simulink model "E33_VCU_simulink"  (R2014a)
settings: Solver=FixedStepDiscrete  StartTime=0.0  StopTime=10.0  FixedStep=0.0005  RelTol=1e-3
values from neighbouring files (symbols this model uses):
  Accu_FAN_Test = ecucoder_cal(Accu_FAN_Test)    [E33_VCU.m]
  Accu_FAN_threshold = ecucoder_cal(Accu_FAN_threshold)    [E33_VCU.m]
  APPS1_Voltage = ecucoder_cal(APPS1_Voltage)    [E33_VCU.m]
  APPS2_Voltage = ecucoder_cal(APPS2_Voltage)    [E33_VCU.m]
  APPS_Map = [0,1000]    [E33_VCU.m]
  APPS_threshold = ecucoder_cal(APPS_threshold)    [E33_VCU.m]
  Beep_Time = ecucoder_cal(Beep_Time)    [E33_VCU.m]
  BeeperTest = ecucoder_cal(BeeperTest)    [E33_VCU.m]
  BMSLedTest = ecucoder_cal(BMSLedTest)    [E33_VCU.m]
  BP_F_threshold = ecucoder_cal(BP_F_threshold)    [E33_VCU.m]
  BP_F_Voltage = ecucoder_cal(BP_F_Voltage)    [E33_VCU.m]
  BP_Map = [0,1000]    [E33_VCU.m]
  BP_R_Voltage = ecucoder_cal(BP_R_Voltage)    [E33_VCU.m]
  Brk_luminance = ecucoder_cal(Brk_luminance)    [E33_VCU.m]
  DCDC_Relay_Test = ecucoder_cal(DCDC_Relay_Test)    [E33_VCU.m]
  FactoryTestEnable = ecucoder_cal(FactoryTestEnable)    [E33_VCU.m]
  HardBrk_luminance = ecucoder_cal(HardBrk_luminance)    [E33_VCU.m]
  IMDLedTest = ecucoder_cal(IMDLedTest)    [E33_VCU.m]
  linear_FL_Map = ecucoder_cal(linear_FL_Map)    [E33_VCU.m]
  linear_FR_Map = ecucoder_cal(linear_FR_Map)    [E33_VCU.m]
  linear_Map = ecucoder_cal(linear_Map)    [E33_VCU.m]
  linear_RL_Map = ecucoder_cal(linear_RL_Map)    [E33_VCU.m]
  linear_RR_Map = ecucoder_cal(linear_RR_Map)    [E33_VCU.m]
  MaxPow = 40    [E33_VCU.m]
  MaxRPM = 5400    [E33_VCU.m]
  MaxRPMchangePerSec = ecucoder_cal(MaxRPMchangePerSec)    [E33_VCU.m]
  MaxTorqChangePerSec = ecucoder_cal(MaxTorqChangePerSec)    [E33_VCU.m]
  Motor_RPM_Map = (0:ceil(MaxRPM/100))*100    [E33_VCU.m]
  Pump_Test = ecucoder_cal(Pump_Test)    [E33_VCU.m]
  Pump_threshold = ecucoder_cal(Pump_threshold)    [E33_VCU.m]
  R2D_Light_Test = ecucoder_cal(R2D_Light_Test)    [E33_VCU.m]
  Radiator_FAN_Test = ecucoder_cal(Radiator_FAN_Test)    [E33_VCU.m]
  SCS_Error_5V = ecucoder_cal(SCS_Error_5V)    [E33_VCU.m]
  SCS_Error_GND = ecucoder_cal(SCS_Error_GND)    [E33_VCU.m]
  SPD_Coef = 1884/40    (= 47.1)    [E33_VCU.m]
  Tail_Light_Test = ecucoder_cal(Tail_Light_Test)    [E33_VCU.m]
  Tmanage_Map = [0,100]    [E33_VCU.m]
  Torq_percentage_Map = Motor_Torq_MAP/MaxTorq*1000    [E33_VCU.m]
libraries: simulink x164, ec55xxlib x44, dspswit3 x6
(part 2 of 5)

== system E33_VCU_simulink/Input/Input/Sensor ==
  function : TriggerPort  TriggerType=function-call
  1-D Lookup Table1 : Lookup_n-D  NumberOfTableDimensions=1  BreakpointsForDimension1=linear_RR_Map  Table=linear_Map  ExtrapMethod=Clip  InternalRulePriority=Speed  OutDataTypeStr=uint16  RndMeth=Simplest  InputSameDT=on
  1-D Lookup Table2 : Lookup_n-D  NumberOfTableDimensions=1  BreakpointsForDimension1=linear_FR_Map  Table=linear_Map  ExtrapMethod=Clip  InternalRulePriority=Speed  OutDataTypeStr=uint16  RndMeth=Simplest  InputSameDT=on
  1-D Lookup Table3 : Lookup_n-D  NumberOfTableDimensions=1  BreakpointsForDimension1=linear_RL_Map  Table=linear_Map  ExtrapMethod=Clip  InternalRulePriority=Speed  OutDataTypeStr=uint16  RndMeth=Simplest  InputSameDT=on
  1-D Lookup Table4 : Lookup_n-D  NumberOfTableDimensions=1  BreakpointsForDimension1=linear_FL_Map  Table=linear_Map  ExtrapMethod=Clip  InternalRulePriority=Speed  OutDataTypeStr=uint16  RndMeth=Simplest  InputSameDT=on
  1-D Lookup Table5 : Lookup_n-D  NumberOfTableDimensions=1  BreakpointsForDimension1=[500,900,2007,2205,3405,3705,4490]  BreakpointsForDimension1DataTypeStr=int32  Table=[-364,0,1000,1000,-1000,-1000,-365]  TableDataTypeStr=int32  IntermediateResultsDataTypeStr=int32  ExtrapMethod=Clip  InternalRulePriority=Speed  OutDataTypeStr=int32  RndMeth=Simplest  InputSameDT=on
  AnalogInput : ec55xxlib/RapidECU_U2/02AnalogInput/AnalogInput  channel=56: I_AN17_5V  sampletime=-1
  AnalogInput1 : ec55xxlib/RapidECU_U2/02AnalogInput/AnalogInput  channel=71: I_AN18_5V  sampletime=-1
  AnalogInput2 : ec55xxlib/RapidECU_U2/02AnalogInput/AnalogInput  channel=73: I_AN19_5V  sampletime=-1
  AnalogInput3 : ec55xxlib/RapidECU_U2/02AnalogInput/AnalogInput  channel=74: I_AN20_5V  sampletime=-1
  AnalogInput4 : ec55xxlib/RapidECU_U2/02AnalogInput/AnalogInput  channel=14: I_AN04_2K55  sampletime=-1
  Constant : Constant  Commented=on  Value=SPD_Coef
  Data Type Conversion{,1..3} (4 alike) : DataTypeConversion  Commented=on  OutDataTypeStr=double
  Demux : Demux  Commented=on
  Filter1 : Subsystem
  Filter2 : Subsystem
  Filter3 : Subsystem
  Filter4 : Subsystem
  For Each Subsystem : Subsystem  Commented=on  TreatAsAtomicUnit=on
  FrequencyRead : ec55xxlib/RapidECU_U2/03FrequencyInput/FrequencyRead  Commented=on  channel=41: I_HALL5  sampletime=-1
  FrequencyRead1 : ec55xxlib/RapidECU_U2/03FrequencyInput/FrequencyRead  Commented=on  channel=38: I_HALL2  sampletime=-1
  FrequencyRead2 : ec55xxlib/RapidECU_U2/03FrequencyInput/FrequencyRead  Commented=on  channel=39: I_HALL3  sampletime=-1
  FrequencyRead3 : ec55xxlib/RapidECU_U2/03FrequencyInput/FrequencyRead  Commented=on  channel=40: I_HALL4  sampletime=-1
  Mux : Mux  Commented=on
  Linear_RR : Outport
  Linear_FR : Outport  Port=2
  Linear_RL : Outport  Port=3
  Linear_FL : Outport  Port=4
  Wheel_Angle : Outport  Port=5
  wires:
  AnalogInput3/1 -> Filter4/1(In)
  AnalogInput2/1 -> Filter2/1(In)
  AnalogInput1/1 -> Filter1/1(In)
  AnalogInput/1 -> Filter3/1(In)
  AnalogInput4/1 -> 1-D Lookup Table5/1  "Angle_Vol"
  Filter3/1(Out) -> 1-D Lookup Table1/1
  1-D Lookup Table1/1 -> Linear_RR/1
  Filter1/1(Out) -> 1-D Lookup Table2/1
  1-D Lookup Table2/1 -> Linear_FR/1
  Filter2/1(Out) -> 1-D Lookup Table3/1
  1-D Lookup Table3/1 -> Linear_RL/1
  Filter4/1(Out) -> 1-D Lookup Table4/1
  1-D Lookup Table4/1 -> Linear_FL/1
  1-D Lookup Table5/1 -> Wheel_Angle/1
  FrequencyRead1/1 -> Mux/1  "SPD_RR_Vol"
  FrequencyRead2/1 -> Mux/2  "SPD_FR_Voll"
  FrequencyRead3/1 -> Mux/3
  FrequencyRead/1 -> Mux/4
  Mux/1 -> For Each Subsystem/1(In1)
  Constant/1 -> For Each Subsystem/2(In2)
  For Each Subsystem/1(Out1) -> Demux/1
  Demux/1 -> Data Type Conversion/1  "SPD_RR"
  Demux/2 -> Data Type Conversion1/1  "SPD_FR"
  Demux/3 -> Data Type Conversion2/1  "SPD_RL"
  Demux/4 -> Data Type Conversion3/1  "SPD_FL"
  Data Type Conversion/1 -> ?
  Data Type Conversion1/1 -> ?
  Data Type Conversion2/1 -> ?
  Data Type Conversion3/1 -> ?

== system E33_VCU_simulink/Subsystem1/MCUctrl/MCU_CMD_CAN_Tx ==
  Msg : Inport
  Enable : EnablePort
  CANTransmit : ec55xxlib/RapidECU_U2/07CANCommucation/CANTransmit  canmodule=A  canbuffer=8  canmessageid=hex2dec('08C1EF21')  canmessagetype=Extended(29-bit ID)  datalength=8  sampletime=-1
  CAN_OK : Outport
  wires:
  Msg/1 -> CANTransmit/1
  CANTransmit/1 -> CAN_OK/1  "VCUMCUCANOKK"

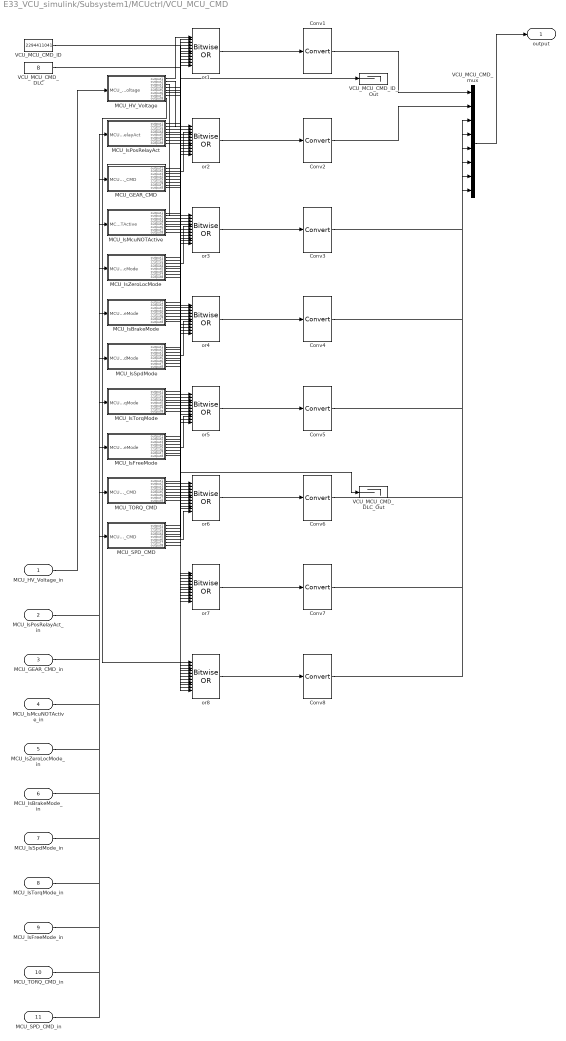
== system E33_VCU_simulink/Subsystem1/MCUctrl/VCU_MCU_CMD ==
  MCU_HV_Voltage_in : Inport
  MCU_IsPosRelayAct_in : Inport  Port=2
  MCU_GEAR_CMD_in : Inport  Port=3
  MCU_IsMcuNOTActive_in : Inport  Port=4
  MCU_IsZeroLocMode_in : Inport  Port=5
  MCU_IsBrakeMode_in : Inport  Port=6
  MCU_IsSpdMode_in : Inport  Port=7
  MCU_IsTorqMode_in : Inport  Port=8
  MCU_IsFreeMode_in : Inport  Port=9
  MCU_TORQ_CMD_in : Inport  Port=10
  MCU_SPD_CMD_in : Inport  Port=11
  Conv{1..8} (8 alike) : DataTypeConversion
  MCU_GEAR_CMD : Subsystem
  MCU_HV_Voltage : Subsystem
  MCU_IsBrakeMode : Subsystem
  MCU_IsFreeMode : Subsystem
  MCU_IsMcuNOTActive : Subsystem
  MCU_IsPosRelayAct : Subsystem
  MCU_IsSpdMode : Subsystem
  MCU_IsTorqMode : Subsystem
  MCU_IsZeroLocMode : Subsystem
  MCU_SPD_CMD : Subsystem
  MCU_TORQ_CMD : Subsystem
  VCU_MCU_CMD_DLC : Constant  Value=8  OutDataTypeStr=uint8
  VCU_MCU_CMD_DLC_Out : Terminator
  VCU_MCU_CMD_ID : Constant  Value=2294411041  OutDataTypeStr=single
  VCU_MCU_CMD_ID_Out : Terminator
  VCU_MCU_CMD_mux : Mux  Inputs=8
  or{1..8} (8 alike) : simulink/Logic and Bit Operations/Bitwise Operator  logicop=OR  UseBitMask=off  NumInputPorts=11  BitMask=bin2dec('11011001')  BitMaskRealWorld=Stored Integer
  output : Outport
  wires:
  VCU_MCU_CMD_mux/1 -> output/1
  MCU_HV_Voltage/1(output1) -> or1/1
  MCU_HV_Voltage/2(output2) -> or2/1
  MCU_HV_Voltage/3(output3) -> or3/1
  MCU_HV_Voltage/4(output4) -> or4/1
  MCU_HV_Voltage/5(output5) -> or5/1
  MCU_HV_Voltage/6(output6) -> or6/1
  MCU_HV_Voltage/7(output7) -> or7/1
  MCU_HV_Voltage/8(output8) -> or8/1
  MCU_IsPosRelayAct/1(output1) -> or1/2
  MCU_IsPosRelayAct/2(output2) -> or2/2
  MCU_IsPosRelayAct/3(output3) -> or3/2
  MCU_IsPosRelayAct/4(output4) -> or4/2
  MCU_IsPosRelayAct/5(output5) -> or5/2
  MCU_IsPosRelayAct/6(output6) -> or6/2
  MCU_IsPosRelayAct/7(output7) -> or7/2
  MCU_IsPosRelayAct/8(output8) -> or8/2
  MCU_GEAR_CMD/1(output1) -> or1/3
  MCU_GEAR_CMD/2(output2) -> or2/3
  MCU_GEAR_CMD/3(output3) -> or3/3
  MCU_GEAR_CMD/4(output4) -> or4/3
  MCU_GEAR_CMD/5(output5) -> or5/3
  MCU_GEAR_CMD/6(output6) -> or6/3
  MCU_GEAR_CMD/7(output7) -> or7/3
  MCU_GEAR_CMD/8(output8) -> or8/3
  MCU_IsMcuNOTActive/1(output1) -> or1/4
  MCU_IsMcuNOTActive/2(output2) -> or2/4
  MCU_IsMcuNOTActive/3(output3) -> or3/4
  MCU_IsMcuNOTActive/4(output4) -> or4/4
  MCU_IsMcuNOTActive/5(output5) -> or5/4
  MCU_IsMcuNOTActive/6(output6) -> or6/4
  MCU_IsMcuNOTActive/7(output7) -> or7/4
  MCU_IsMcuNOTActive/8(output8) -> or8/4
  MCU_IsZeroLocMode/1(output1) -> or1/5
  MCU_IsZeroLocMode/2(output2) -> or2/5
  MCU_IsZeroLocMode/3(output3) -> or3/5
  MCU_IsZeroLocMode/4(output4) -> or4/5
  MCU_IsZeroLocMode/5(output5) -> or5/5
  MCU_IsZeroLocMode/6(output6) -> or6/5
  MCU_IsZeroLocMode/7(output7) -> or7/5
  MCU_IsZeroLocMode/8(output8) -> or8/5
  MCU_IsBrakeMode/1(output1) -> or1/6
  MCU_IsBrakeMode/2(output2) -> or2/6
  MCU_IsBrakeMode/3(output3) -> or3/6
  MCU_IsBrakeMode/4(output4) -> or4/6
  MCU_IsBrakeMode/5(output5) -> or5/6
  MCU_IsBrakeMode/6(output6) -> or6/6
  MCU_IsBrakeMode/7(output7) -> or7/6
  MCU_IsBrakeMode/8(output8) -> or8/6
  MCU_IsSpdMode/1(output1) -> or1/7
  MCU_IsSpdMode/2(output2) -> or2/7
  MCU_IsSpdMode/3(output3) -> or3/7
  MCU_IsSpdMode/4(output4) -> or4/7
  MCU_IsSpdMode/5(output5) -> or5/7
  MCU_IsSpdMode/6(output6) -> or6/7
  MCU_IsSpdMode/7(output7) -> or7/7
  MCU_IsSpdMode/8(output8) -> or8/7
  MCU_IsTorqMode/1(output1) -> or1/8
  MCU_IsTorqMode/2(output2) -> or2/8
  MCU_IsTorqMode/3(output3) -> or3/8
  MCU_IsTorqMode/4(output4) -> or4/8
  MCU_IsTorqMode/5(output5) -> or5/8
  MCU_IsTorqMode/6(output6) -> or6/8
  MCU_IsTorqMode/7(output7) -> or7/8
  MCU_IsTorqMode/8(output8) -> or8/8
  MCU_IsFreeMode/1(output1) -> or1/9
  MCU_IsFreeMode/2(output2) -> or2/9
  MCU_IsFreeMode/3(output3) -> or3/9
  MCU_IsFreeMode/4(output4) -> or4/9
  MCU_IsFreeMode/5(output5) -> or5/9
  MCU_IsFreeMode/6(output6) -> or6/9
  MCU_IsFreeMode/7(output7) -> or7/9
  MCU_IsFreeMode/8(output8) -> or8/9
  MCU_TORQ_CMD/1(output1) -> or1/10
  MCU_TORQ_CMD/2(output2) -> or2/10
  MCU_TORQ_CMD/3(output3) -> or3/10
  MCU_TORQ_CMD/4(output4) -> or4/10
  MCU_TORQ_CMD/5(output5) -> or5/10
  MCU_TORQ_CMD/6(output6) -> or6/10
  MCU_TORQ_CMD/7(output7) -> or7/10
  MCU_TORQ_CMD/8(output8) -> or8/10
  MCU_SPD_CMD/1(output1) -> or1/11
  MCU_SPD_CMD/2(output2) -> or2/11
  MCU_SPD_CMD/3(output3) -> or3/11
  MCU_SPD_CMD/4(output4) -> or4/11
  MCU_SPD_CMD/5(output5) -> or5/11
  MCU_SPD_CMD/6(output6) -> or6/11
  MCU_SPD_CMD/7(output7) -> or7/11
  MCU_SPD_CMD/8(output8) -> or8/11
  or1/1 -> Conv1/1
  Conv1/1 -> VCU_MCU_CMD_mux/1
  or2/1 -> Conv2/1
  Conv2/1 -> VCU_MCU_CMD_mux/2
  or3/1 -> Conv3/1
  Conv3/1 -> VCU_MCU_CMD_mux/3
  or4/1 -> Conv4/1
  Conv4/1 -> VCU_MCU_CMD_mux/4
  or5/1 -> Conv5/1
  Conv5/1 -> VCU_MCU_CMD_mux/5
  or6/1 -> Conv6/1
  Conv6/1 -> VCU_MCU_CMD_mux/6
  or7/1 -> Conv7/1
  Conv7/1 -> VCU_MCU_CMD_mux/7
  or8/1 -> Conv8/1
  Conv8/1 -> VCU_MCU_CMD_mux/8
  VCU_MCU_CMD_ID/1 -> VCU_MCU_CMD_ID_Out/1
  VCU_MCU_CMD_DLC/1 -> VCU_MCU_CMD_DLC_Out/1
  MCU_HV_Voltage_in/1 -> MCU_HV_Voltage/1(MCU_HV_Voltage)
  MCU_IsPosRelayAct_in/1 -> MCU_IsPosRelayAct/1(MCU_IsPosRelayAct)
  MCU_GEAR_CMD_in/1 -> MCU_GEAR_CMD/1(MCU_GEAR_CMD)
  MCU_IsMcuNOTActive_in/1 -> MCU_IsMcuNOTActive/1(MCU_IsMcuNOTActive)
  MCU_IsZeroLocMode_in/1 -> MCU_IsZeroLocMode/1(MCU_IsZeroLocMode)
  MCU_IsBrakeMode_in/1 -> MCU_IsBrakeMode/1(MCU_IsBrakeMode)
  MCU_IsSpdMode_in/1 -> MCU_IsSpdMode/1(MCU_IsSpdMode)
  MCU_IsTorqMode_in/1 -> MCU_IsTorqMode/1(MCU_IsTorqMode)
  MCU_IsFreeMode_in/1 -> MCU_IsFreeMode/1(MCU_IsFreeMode)
  MCU_TORQ_CMD_in/1 -> MCU_TORQ_CMD/1(MCU_TORQ_CMD)
  MCU_SPD_CMD_in/1 -> MCU_SPD_CMD/1(MCU_SPD_CMD)

== system E33_VCU_simulink/Subsystem1/VCUCAN/VCU_Panel ==
  Wheel_Angle_in : Inport
  Linear_RR_in : Inport  Port=2
  Linear_FR_in : Inport  Port=3
  Linear_RL_in : Inport  Port=4
  Linear_FL_in : Inport  Port=5
  Conv{1..8} (8 alike) : DataTypeConversion
  Linear_FL : Subsystem
  Linear_FR : Subsystem
  Linear_RL : Subsystem
  Linear_RR : Subsystem
  VCU_Panel_DLC : Constant  Value=8  OutDataTypeStr=uint8
  VCU_Panel_DLC_Out : Terminator
  VCU_Panel_ID : Constant  Value=2533359616  OutDataTypeStr=single
  VCU_Panel_ID_Out : Terminator
  VCU_Panel_mux : Mux  Inputs=8
  Wheel_Angle : Subsystem
  or{1..8} (8 alike) : simulink/Logic and Bit Operations/Bitwise Operator  logicop=OR  UseBitMask=off  NumInputPorts=5  BitMask=bin2dec('11011001')  BitMaskRealWorld=Stored Integer
  output : Outport
  wires:
  VCU_Panel_mux/1 -> output/1
  Wheel_Angle/1(output1) -> or1/1
  Wheel_Angle/2(output2) -> or2/1
  Wheel_Angle/3(output3) -> or3/1
  Wheel_Angle/4(output4) -> or4/1
  Wheel_Angle/5(output5) -> or5/1
  Wheel_Angle/6(output6) -> or6/1
  Wheel_Angle/7(output7) -> or7/1
  Wheel_Angle/8(output8) -> or8/1
  Linear_RR/1(output1) -> or1/2
  Linear_RR/2(output2) -> or2/2
  Linear_RR/3(output3) -> or3/2
  Linear_RR/4(output4) -> or4/2
  Linear_RR/5(output5) -> or5/2
  Linear_RR/6(output6) -> or6/2
  Linear_RR/7(output7) -> or7/2
  Linear_RR/8(output8) -> or8/2
  Linear_FR/1(output1) -> or1/3
  Linear_FR/2(output2) -> or2/3
  Linear_FR/3(output3) -> or3/3
  Linear_FR/4(output4) -> or4/3
  Linear_FR/5(output5) -> or5/3
  Linear_FR/6(output6) -> or6/3
  Linear_FR/7(output7) -> or7/3
  Linear_FR/8(output8) -> or8/3
  Linear_RL/1(output1) -> or1/4
  Linear_RL/2(output2) -> or2/4
  Linear_RL/3(output3) -> or3/4
  Linear_RL/4(output4) -> or4/4
  Linear_RL/5(output5) -> or5/4
  Linear_RL/6(output6) -> or6/4
  Linear_RL/7(output7) -> or7/4
  Linear_RL/8(output8) -> or8/4
  Linear_FL/1(output1) -> or1/5
  Linear_FL/2(output2) -> or2/5
  Linear_FL/3(output3) -> or3/5
  Linear_FL/4(output4) -> or4/5
  Linear_FL/5(output5) -> or5/5
  Linear_FL/6(output6) -> or6/5
  Linear_FL/7(output7) -> or7/5
  Linear_FL/8(output8) -> or8/5
  or1/1 -> Conv1/1
  Conv1/1 -> VCU_Panel_mux/1
  or2/1 -> Conv2/1
  Conv2/1 -> VCU_Panel_mux/2
  or3/1 -> Conv3/1
  Conv3/1 -> VCU_Panel_mux/3
  or4/1 -> Conv4/1
  Conv4/1 -> VCU_Panel_mux/4
  or5/1 -> Conv5/1
  Conv5/1 -> VCU_Panel_mux/5
  or6/1 -> Conv6/1
  Conv6/1 -> VCU_Panel_mux/6
  or7/1 -> Conv7/1
  Conv7/1 -> VCU_Panel_mux/7
  or8/1 -> Conv8/1
  Conv8/1 -> VCU_Panel_mux/8
  VCU_Panel_ID/1 -> VCU_Panel_ID_Out/1
  VCU_Panel_DLC/1 -> VCU_Panel_DLC_Out/1
  Wheel_Angle_in/1 -> Wheel_Angle/1(Wheel_Angle)
  Linear_RR_in/1 -> Linear_RR/1(Linear_RR)
  Linear_FR_in/1 -> Linear_FR/1(Linear_FR)
  Linear_RL_in/1 -> Linear_RL/1(Linear_RL)
  Linear_FL_in/1 -> Linear_FL/1(Linear_FL)

== system E33_VCU_simulink/Input/Input/APPS/Filter1  ==
  In : Inport
  Add : Sum  Inputs=-+-
  Constant : Constant  Value=4  OutDataTypeStr=uint8  SampleTime=-1
  Divide : Product  Inputs=*/
  MinMax : MinMax
  MinMax1 : MinMax  Function=max
  Sum of Elements : Sum  Inputs=+
  Tapped Delay : simulink/Discrete/Tapped Delay  vinit=0  samptime=-1  NumDelays=6  DelayOrder=Oldest  includeCurrent=off
  Out : Outport
  wires:
  Constant/1 -> Divide/2
  Sum of Elements/1 -> Add/2
  MinMax1/1 -> Add/1
  MinMax/1 -> Add/3
  Add/1 -> Divide/1
  In/1 -> Tapped Delay/1
  Divide/1 -> Out/1
  Tapped Delay/1 -> Sum of Elements/1, MinMax1/1, MinMax/1

== system E33_VCU_simulink/Input/Input/APPS/Filter2  ==
  In : Inport
  Add : Sum  Inputs=-+-
  Constant : Constant  Value=4  OutDataTypeStr=uint8  SampleTime=-1
  Divide : Product  Inputs=*/
  MinMax : MinMax
  MinMax1 : MinMax  Function=max
  Sum of Elements : Sum  Inputs=+
  Tapped Delay : simulink/Discrete/Tapped Delay  vinit=0  samptime=-1  NumDelays=6  DelayOrder=Oldest  includeCurrent=off
  Out : Outport
  wires:
  Constant/1 -> Divide/2
  Sum of Elements/1 -> Add/2
  MinMax1/1 -> Add/1
  MinMax/1 -> Add/3
  Add/1 -> Divide/1
  In/1 -> Tapped Delay/1
  Divide/1 -> Out/1
  Tapped Delay/1 -> Sum of Elements/1, MinMax1/1, MinMax/1

== system E33_VCU_simulink/Input/Input/APPS/Reliability testing ==
  APPS1_Pos : Inport
  APPS2_Pos : Inport  Port=2
  Constant : Constant  Value=1000
  Difference in pedal travel : Sum  Inputs=+-  OutDataTypeStr=uint16
  Pedal stroke 10% : simulink/Logic and Bit Operations/Compare To Constant  relop=>=  const=1100  OutDataTypeStr=uint8
  Sum : Sum  Inputs=|++
  APPS_Unreliable : Outport
  wires:
  APPS1_Pos/1 -> Sum/1
  Difference in pedal travel/1 -> Pedal stroke 10%/1  "APPSUn_dif"
  Pedal stroke 10%/1 -> APPS_Unreliable/1
  Sum/1 -> Difference in pedal travel/1
  APPS2_Pos/1 -> Difference in pedal travel/2
  Constant/1 -> Sum/2

== system E33_VCU_simulink/Input/Input/APPS/SCS_Wire_breakage_detection ==
  APPS1_Voltage : Inport
  APPS2_Voltage : Inport  Port=2
  Compare To Constant : simulink/Logic and Bit Operations/Compare To Constant  relop=>=  const=SCS_Error_5V  OutDataTypeStr=boolean
  Compare To Constant1 : simulink/Logic and Bit Operations/Compare To Constant  relop=<=  const=SCS_Error_GND  OutDataTypeStr=boolean
  Compare To Constant2 : simulink/Logic and Bit Operations/Compare To Constant  relop=>=  const=SCS_Error_5V  OutDataTypeStr=boolean
  Compare To Constant3 : simulink/Logic and Bit Operations/Compare To Constant  relop=<=  const=SCS_Error_GND  OutDataTypeStr=boolean
  Logical Operator : Logic  Operator=OR  AllPortsSameDT=off  OutDataTypeStr=boolean
  Logical Operator1 : Logic  Operator=OR  AllPortsSameDT=off  OutDataTypeStr=boolean
  APPS1_Disconnect : Outport
  APPS2_Disconnect : Outport  Port=2
  wires:
  APPS1_Voltage/1 -> Compare To Constant1/1, Compare To Constant/1
  Compare To Constant1/1 -> Logical Operator/2
  Logical Operator/1 -> APPS1_Disconnect/1
  Compare To Constant/1 -> Logical Operator/1
  APPS2_Voltage/1 -> Compare To Constant3/1, Compare To Constant2/1
  Compare To Constant3/1 -> Logical Operator1/2
  Logical Operator1/1 -> APPS2_Disconnect/1
  Compare To Constant2/1 -> Logical Operator1/1

== system E33_VCU_simulink/Input/Input/APPS/Subsystem ==
  APPS1_Pos : Inport
  APPS2_Pos : Inport  Port=2
  Add : Sum
  Gain : Gain  Gain=0.5
  APPS_Pos : Outport
  wires:
  APPS1_Pos/1 -> Add/1
  Gain/1 -> APPS_Pos/1
  Add/1 -> Gain/1
  APPS2_Pos/1 -> Add/2

== system E33_VCU_simulink/Input/Input/BMS_CAN_Receive/BMS_ALM_Analyze ==
  CAN_OK : Inport
  Msg : Inport  Port=2
  function : TriggerPort  TriggerType=function-call
  Bus Creator : BusCreator  Inputs=25
  Enabled Subsystem : Subsystem  TreatAsAtomicUnit=on
  MsgBus : Outport
  wires:
  Bus Creator/1 -> MsgBus/1
  CAN_OK/1 -> Enabled Subsystem/Enable
  Msg/1 -> Enabled Subsystem/1(input)
  Enabled Subsystem/1(BMS_ALM_VCU_OFFLINE_Out) -> Bus Creator/1  "VCU_OFFLINE"
  Enabled Subsystem/2(BMS_ALM_PRECHG_FAIL_Out) -> Bus Creator/2  "PRECHG_FAIL"
  Enabled Subsystem/3(BMS_ALM_LEAK_OC_Out) -> Bus Creator/3  "LEAK_OC"
  Enabled Subsystem/4(BMS_ALM_HVREL_FAIL_Out) -> Bus Creator/4  "HVREL_FAIL"
  Enabled Subsystem/5(BMS_ALM_HALL_BREAK_Out) -> Bus Creator/5  "HALL_BREAK"
  Enabled Subsystem/6(BMS_ALM_DSCH_OCT_Out) -> Bus Creator/6  "DSCH_OCT"
  Enabled Subsystem/7(BMS_ALM_DSCH_OCS_Out) -> Bus Creator/7  "DSCH_OCS"
  Enabled Subsystem/8(BMS_ALM_CHRG_OCT_Out) -> Bus Creator/8  "CHRG_OCT"
  Enabled Subsystem/9(BMS_ALM_CHRG_OCS_Out) -> Bus Creator/9  "CHRG_OCS"
  Enabled Subsystem/10(BMS_ALM_CELL_UV_Out) -> Bus Creator/10  "CELL_UV"
  Enabled Subsystem/11(BMS_ALM_CELL_UT_Out) -> Bus Creator/11  "CELL_UT"
  Enabled Subsystem/12(BMS_ALM_CELL_TBK_Out) -> Bus Creator/12  "CELL_TBK"
  Enabled Subsystem/13(BMS_ALM_CELL_OV_Out) -> Bus Creator/13  "CELL_OV"
  Enabled Subsystem/14(BMS_ALM_CELL_OT_Out) -> Bus Creator/14  "CELL_OT"
  Enabled Subsystem/15(BMS_ALM_CELL_LBK_Out) -> Bus Creator/15  "CELL_LBK"
  Enabled Subsystem/16(BMS_ALM_CELL_DV_Out) -> Bus Creator/16  "CELL_DV"
  Enabled Subsystem/17(BMS_ALM_CELL_DT_Out) -> Bus Creator/17  "CELL_DT"
  Enabled Subsystem/18(BMS_ALM_BSU_OFFLINE_Out) -> Bus Creator/18  "BSU_OFFLINE"
  Enabled Subsystem/19(BMS_ALM_BSU_FAULT_Out) -> Bus Creator/19  "BSU_FAULT"
  Enabled Subsystem/20(BMS_ALM_BMU_FAIL_Out) -> Bus Creator/20  "BMU_FAIL"
  Enabled Subsystem/21(BMS_ALM_BATT_UV_Out) -> Bus Creator/21  "BATT_UV"
  Enabled Subsystem/22(BMS_ALM_BATT_UC_Out) -> Bus Creator/22  "BAT_UC"
  Enabled Subsystem/23(BMS_ALM_BATT_OV_Out) -> Bus Creator/23  "BATT_OV"
  Enabled Subsystem/24(BMS_ALM_BATT_OC_Out) -> Bus Creator/24  "BATT_OC"
  Enabled Subsystem/25(BMS_ALM_AUX_FAIL_Out) -> Bus Creator/25  "AUX_FAIL"

== system E33_VCU_simulink/Input/Input/BMS_CAN_Receive/BMS_ALM_Analyze1 ==
  CAN_OK : Inport
  Msg : Inport  Port=2
  function : TriggerPort  TriggerType=function-call
  BMS_HCU_MAXV : Subsystem
  Bus Creator : BusCreator
  MsgBus : Outport
  wires:
  Bus Creator/1 -> MsgBus/1
  CAN_OK/1 -> BMS_HCU_MAXV/Enable
  Msg/1 -> BMS_HCU_MAXV/1(input)
  BMS_HCU_MAXV/1(MinCellVoltNo_Out) -> Bus Creator/1  "MinCellVoltNo_Out"
  BMS_HCU_MAXV/2(MaxCellVoltNo_Out) -> Bus Creator/2  "MaxCellVoltNo_Out"
  BMS_HCU_MAXV/3(MinCellVolt_Out) -> Bus Creator/3  "MinCellVolt_Out"
  BMS_HCU_MAXV/4(MaxCellVolt_Out) -> Bus Creator/4  "MaxCellVolt_Out"

== system E33_VCU_simulink/Input/Input/BMS_CAN_Receive/BMS_INFO_Analyze ==
  CAN_OK : Inport
  Msg : Inport  Port=2
  function : TriggerPort  TriggerType=function-call
  Bus Creator : BusCreator  Inputs=7
  Enabled Subsystem : Subsystem  TreatAsAtomicUnit=on
  MsgBus : Outport
  wires:
  Msg/1 -> Enabled Subsystem/1(In1)
  CAN_OK/1 -> Enabled Subsystem/Enable
  Enabled Subsystem/3(Stat) -> Bus Creator/3  "BMS_Stat"
  Enabled Subsystem/2(AlmLv) -> Bus Creator/2  "BMS_AlmLv"
  Enabled Subsystem/4(SoH) -> Bus Creator/4  "BMS_SoH"
  Enabled Subsystem/7(Voltage) -> Bus Creator/7  "BMS_Voltage"
  Enabled Subsystem/1(BatLife) -> Bus Creator/1  "BMS_Life"
  Enabled Subsystem/5(BatSoc) -> Bus Creator/5  "BMS_SoC"
  Enabled Subsystem/6(Current) -> Bus Creator/6  "BMS_Current"
  Bus Creator/1 -> MsgBus/1

== system E33_VCU_simulink/Input/Input/BMS_CAN_Receive/BMS_MAXT_Analyze ==
  CAN_OK : Inport
  Msg : Inport  Port=2
  function : TriggerPort  TriggerType=function-call
  Bus Creator : BusCreator  Inputs=6
  Enabled Subsystem : Subsystem  TreatAsAtomicUnit=on
  MsgBus : Outport
  wires:
  Msg/1 -> Enabled Subsystem/1(input)
  CAN_OK/1 -> Enabled Subsystem/Enable
  Bus Creator/1 -> MsgBus/1
  Enabled Subsystem/1(HeatingCtl_Out) -> Bus Creator/1  "HeatCtrl"
  Enabled Subsystem/4(MaxTempNo_Out) -> Bus Creator/4  "MaxTempNo"
  Enabled Subsystem/5(MinTemp_Out) -> Bus Creator/5  "MinTemp"
  Enabled Subsystem/6(MaxTemp_Out) -> Bus Creator/6  "MaxTemp"
  Enabled Subsystem/2(CoolingCtl_Out) -> Bus Creator/2  "CoolCtrl"
  Enabled Subsystem/3(MinTempNo_Out) -> Bus Creator/3  "MinTempNo"

== system E33_VCU_simulink/Input/Input/Bpressure/SCS_Wire_breakage_detection ==
  BP_F_Voltage : Inport
  BP_R_Voltage : Inport  Port=2
  Compare To Constant : simulink/Logic and Bit Operations/Compare To Constant  relop=>=  const=SCS_Error_5V  OutDataTypeStr=boolean
  Compare To Constant1 : simulink/Logic and Bit Operations/Compare To Constant  relop=<=  const=SCS_Error_GND  OutDataTypeStr=boolean
  Compare To Constant2 : simulink/Logic and Bit Operations/Compare To Constant  relop=>=  const=SCS_Error_5V  OutDataTypeStr=boolean
  Compare To Constant3 : simulink/Logic and Bit Operations/Compare To Constant  relop=<=  const=SCS_Error_GND  OutDataTypeStr=boolean
  Logical Operator : Logic  Operator=OR  AllPortsSameDT=off  OutDataTypeStr=boolean
  Logical Operator1 : Logic  Operator=OR  AllPortsSameDT=off  OutDataTypeStr=boolean
  BP_F_Disconnect : Outport
  BP_R_Disconnect : Outport  Port=2
  wires:
  BP_F_Voltage/1 -> Compare To Constant1/1, Compare To Constant/1
  Compare To Constant1/1 -> Logical Operator/2
  Logical Operator/1 -> BP_F_Disconnect/1
  Compare To Constant/1 -> Logical Operator/1
  BP_R_Voltage/1 -> Compare To Constant3/1, Compare To Constant2/1
  Compare To Constant3/1 -> Logical Operator1/2
  Logical Operator1/1 -> BP_R_Disconnect/1
  Compare To Constant2/1 -> Logical Operator1/1

== system E33_VCU_simulink/Input/Input/Keys/BoolFilter6 ==
  Raw : Inport
  Filtered : Outport
  wires:
  Raw/1 -> Filtered/1

== system E33_VCU_simulink/Input/Input/MCU_CAN_Receive/ReceiveMessages ==
  CAN_OK : Inport
  Msg : Inport  Port=2
  function : TriggerPort  TriggerType=function-call
  Bus Creator : BusCreator  Inputs=20
  MCU_Stat : Subsystem
  CAN_MCU_Stat : Outport
  wires:
  CAN_OK/1 -> MCU_Stat/Enable
  Msg/1 -> MCU_Stat/1(input)
  MCU_Stat/2(MCU_IsSelfcheckPass_Out) -> Bus Creator/2  "MCU_IsSelfcheckPass"
  MCU_Stat/3(MCU_IsMotorOvertemp_Out) -> Bus Creator/3  "MCU_IsMotorOvertemp"
  MCU_Stat/4(MCU_IsMcuOvertemp_Out) -> Bus Creator/4  "MCU_IsMcu_OverTemp"
  MCU_Stat/1(MCU_AlmLv_Out) -> Bus Creator/1  "MCU_AlmLv"
  MCU_Stat/5(MCU_IsUnderPowerLim_Out) -> Bus Creator/5  "MCU_IsUnderPowerLim"
  MCU_Stat/6(MCU_IsHvUndervoltage_Out) -> Bus Creator/6  "MCU_IsHvUndervoltage"
  MCU_Stat/11(MCU_IsPreChg_Out) -> Bus Creator/11  "MCU_IsPreChg"
  MCU_Stat/7(MCU_IsLvError_Out) -> Bus Creator/7  "MCU_IsLvError"
  MCU_Stat/8(MCU_IsHvOvervoltage_Out) -> Bus Creator/8  "MCU_IsHvOverVoltage"
  MCU_Stat/10(MCU_IsRevoloverError_Out) -> Bus Creator/10  "MCU_IsRevloverError"
  MCU_Stat/13(MCU_IsMcuNOTActive_Out) -> Bus Creator/13  "MCU_IsDeactived"
  MCU_Stat/14(MCU_IsZeroLocMode_Out) -> Bus Creator/14  "MCU_IsZeroLocMode"
  MCU_Stat/12(MCU_IsReady_Out) -> Bus Creator/12  "MCU_IsReady"
  MCU_Stat/9(MCU_IsOverCurr_Out) -> Bus Creator/9  "MCU_IsOverCurr"
  MCU_Stat/17(MCU_IsTorqMode_Out) -> Bus Creator/17  "MCU_IsTorqMode"
  MCU_Stat/18(MCU_IsFreeMode_Out) -> Bus Creator/18  "MCU_IsFreeMode"
  MCU_Stat/20(MCU_SPD_RPT_Out) -> Bus Creator/20  "MCU_Spd"
  MCU_Stat/15(MCU_IsBrakeMode_Out) -> Bus Creator/15  "MCU_IsBrakeMode"
  MCU_Stat/16(MCU_IsSpdMode_Out) -> Bus Creator/16  "MCU_IsSpdMode"
  MCU_Stat/19(MCU_TORQ_RPT_Out) -> Bus Creator/19  "MCU_Torq"
  Bus Creator/1 -> CAN_MCU_Stat/1

== system E33_VCU_simulink/Input/Input/MCU_CAN_Receive/ReceiveMessages1 ==
  CAN_OK : Inport
  Msg : Inport  Port=2
  function : TriggerPort  TriggerType=function-call
  Bus Creator1 : BusCreator  Inputs=5
  Enabled Subsystem : Subsystem  TreatAsAtomicUnit=on
  CAN_MCU_Pwr : Outport
  wires:
  Enabled Subsystem/2(MCU_HvCurr_Out) -> Bus Creator1/2  "MCU_HvDcCurr"
  Enabled Subsystem/3(MCU_HvVolt_Out) -> Bus Creator1/3  "MCU_HvVolt"
  Enabled Subsystem/1(MCU_HvAcCurrRms_Out) -> Bus Creator1/1  "MCU_HvAcCurrRMS"
  Enabled Subsystem/4(MCU_MotorTemp_Out) -> Bus Creator1/4  "MCU_MotorTemp"
  Enabled Subsystem/5(MCU_McuTemp_Out) -> Bus Creator1/5  "MCU_McuTemp"
  Bus Creator1/1 -> CAN_MCU_Pwr/1
  Msg/1 -> Enabled Subsystem/1(input)
  CAN_OK/1 -> Enabled Subsystem/Enable

== system E33_VCU_simulink/Input/Input/Sensor/Filter1 ==
  In : Inport
  Add : Sum  Inputs=-+-
  Constant : Constant  Value=4  OutDataTypeStr=uint8  SampleTime=-1
  Divide : Product  Inputs=*/
  MinMax : MinMax
  MinMax1 : MinMax  Function=max
  Sum of Elements : Sum  Inputs=+
  Tapped Delay : simulink/Discrete/Tapped Delay  vinit=0  samptime=-1  NumDelays=6  DelayOrder=Oldest  includeCurrent=off
  Out : Outport
  wires:
  Constant/1 -> Divide/2
  Sum of Elements/1 -> Add/2
  MinMax1/1 -> Add/1
  MinMax/1 -> Add/3
  Add/1 -> Divide/1
  In/1 -> Tapped Delay/1
  Divide/1 -> Out/1
  Tapped Delay/1 -> Sum of Elements/1, MinMax1/1, MinMax/1

== system E33_VCU_simulink/Input/Input/Sensor/Filter2 ==
  In : Inport
  Add : Sum  Inputs=-+-
  Constant : Constant  Value=4  OutDataTypeStr=uint8  SampleTime=-1
  Divide : Product  Inputs=*/
  MinMax : MinMax
  MinMax1 : MinMax  Function=max
  Sum of Elements : Sum  Inputs=+
  Tapped Delay : simulink/Discrete/Tapped Delay  vinit=0  samptime=-1  NumDelays=6  DelayOrder=Oldest  includeCurrent=off
  Out : Outport
  wires:
  Constant/1 -> Divide/2
  Sum of Elements/1 -> Add/2
  MinMax1/1 -> Add/1
  MinMax/1 -> Add/3
  Add/1 -> Divide/1
  In/1 -> Tapped Delay/1
  Divide/1 -> Out/1
  Tapped Delay/1 -> Sum of Elements/1, MinMax1/1, MinMax/1

== system E33_VCU_simulink/Input/Input/Sensor/Filter3 ==
  In : Inport
  Add : Sum  Inputs=-+-
  Constant : Constant  Value=4  OutDataTypeStr=uint8  SampleTime=-1
  Divide : Product  Inputs=*/
  MinMax : MinMax
  MinMax1 : MinMax  Function=max
  Sum of Elements : Sum  Inputs=+
  Tapped Delay : simulink/Discrete/Tapped Delay  vinit=0  samptime=-1  NumDelays=6  DelayOrder=Oldest  includeCurrent=off
  Out : Outport
  wires:
  Constant/1 -> Divide/2
  Sum of Elements/1 -> Add/2
  MinMax1/1 -> Add/1
  MinMax/1 -> Add/3
  Add/1 -> Divide/1
  In/1 -> Tapped Delay/1
  Divide/1 -> Out/1
  Tapped Delay/1 -> Sum of Elements/1, MinMax1/1, MinMax/1

== system E33_VCU_simulink/Input/Input/Sensor/Filter4 ==
  In : Inport
  Add : Sum  Inputs=-+-
  Constant : Constant  Value=4  OutDataTypeStr=uint8  SampleTime=-1
  Divide : Product  Inputs=*/
  MinMax : MinMax
  MinMax1 : MinMax  Function=max
  Sum of Elements : Sum  Inputs=+
  Tapped Delay : simulink/Discrete/Tapped Delay  vinit=0  samptime=-1  NumDelays=6  DelayOrder=Oldest  includeCurrent=off
  Out : Outport
  wires:
  Constant/1 -> Divide/2
  Sum of Elements/1 -> Add/2
  MinMax1/1 -> Add/1
  MinMax/1 -> Add/3
  Add/1 -> Divide/1
  In/1 -> Tapped Delay/1
  Divide/1 -> Out/1
  Tapped Delay/1 -> Sum of Elements/1, MinMax1/1, MinMax/1

== system E33_VCU_simulink/Input/Input/Sensor/For Each Subsystem ==
  In1 : Inport  Partition=on  PartitionDimension=1  PartitionWidth=1
  In2 : Inport  Port=2  Partition=off
  Filter5 : Subsystem  Commented=on
  For Each : ForEach  DisableCoverage=on  IndexMode=One-based
  Product : Product
  Out1 : Outport  ConcatenationDimension=1
  wires:
  In1/1 -> Product/2
  In2/1 -> Product/1
  Product/1 -> Out1/1

== system E33_VCU_simulink/Subsystem1/MCUctrl/VCU_MCU_CMD/MCU_GEAR_CMD ==
  MCU_GEAR_CMD : Inport
  Constant{1..5,7..8} (7 alike) : Constant  Value=0  OutDataTypeStr=uint8  SampleTime=-1
  MCU_GEAR_CMDRon : Rounding  Operator=round
  MCU_GEAR_CMD_1sat : Saturate  UpperLimit=3  LowerLimit=0
  MCU_GEAR_CMD_Convert : DataTypeConversion  OutDataTypeStr=uint8
  MCU_GEAR_CMD_Convert1 : DataTypeConversion  OutDataTypeStr=uint32
  MCU_GEAR_CMD_D : Product  Inputs=*/
  MCU_GEAR_CMD_F : Constant  OutDataTypeStr=single
  MCU_GEAR_CMD_L : simulink/Logic and Bit Operations/Bitwise Operator  logicop=AND  UseBitMask=on  BitMask=3  BitMaskRealWorld=Stored Integer
  MCU_GEAR_CMD_O : Constant  Value=0  OutDataTypeStr=single
  MCU_GEAR_CMD_S : ArithShift
  MCU_GEAR_CMD_sat : Saturate  UpperLimit=3  LowerLimit=0
  MCU_GEAR_CMD_st : Sum  Inputs=+-
  output1 : Outport
  output2 : Outport  Port=2
  output3 : Outport  Port=3
  output4 : Outport  Port=4
  output5 : Outport  Port=5
  output6 : Outport  Port=6
  output7 : Outport  Port=7
  output8 : Outport  Port=8
  wires:
  MCU_GEAR_CMD/1 -> MCU_GEAR_CMD_sat/1
  MCU_GEAR_CMD_sat/1 -> MCU_GEAR_CMD_st/1
  MCU_GEAR_CMD_O/1 -> MCU_GEAR_CMD_st/2
  MCU_GEAR_CMD_st/1 -> MCU_GEAR_CMD_D/1
  MCU_GEAR_CMD_F/1 -> MCU_GEAR_CMD_D/2
  MCU_GEAR_CMD_D/1 -> MCU_GEAR_CMDRon/1
  MCU_GEAR_CMDRon/1 -> MCU_GEAR_CMD_S/1
  MCU_GEAR_CMD_S/1 -> MCU_GEAR_CMD_1sat/1
  MCU_GEAR_CMD_1sat/1 -> MCU_GEAR_CMD_Convert1/1
  MCU_GEAR_CMD_Convert1/1 -> MCU_GEAR_CMD_L/1
  MCU_GEAR_CMD_L/1 -> MCU_GEAR_CMD_Convert/1
  MCU_GEAR_CMD_Convert/1 -> output6/1
  Constant1/1 -> output1/1
  Constant2/1 -> output2/1
  Constant3/1 -> output3/1
  Constant4/1 -> output4/1
  Constant5/1 -> output5/1
  Constant7/1 -> output7/1
  Constant8/1 -> output8/1

== system E33_VCU_simulink/Subsystem1/MCUctrl/VCU_MCU_CMD/MCU_HV_Voltage ==
  MCU_HV_Voltage : Inport
  BitCov : DataTypeConversion  OutDataTypeStr=uint8
  Constant{1..6} (6 alike) : Constant  Value=0  OutDataTypeStr=uint8  SampleTime=-1
  MCU_HV_VoltageCOV : DataTypeConversion  OutDataTypeStr=uint8
  MCU_HV_VoltageRon : Rounding  Operator=round
  MCU_HV_Voltage_1sat : Saturate  UpperLimit=65535  LowerLimit=0
  MCU_HV_Voltage_And : simulink/Logic and Bit Operations/Bitwise Operator  logicop=AND  UseBitMask=off  NumInputPorts=2  BitMask=bin2dec('11011001')  BitMaskRealWorld=Stored Integer
  MCU_HV_Voltage_And_C : Constant  Value=255  OutDataTypeStr=uint32
  MCU_HV_Voltage_Convert : DataTypeConversion  OutDataTypeStr=uint32
  MCU_HV_Voltage_D : Product  Inputs=*/
  MCU_HV_Voltage_D1 : Product  Inputs=*/
  MCU_HV_Voltage_F : Constant  Value=0.1  OutDataTypeStr=single
  MCU_HV_Voltage_L : simulink/Logic and Bit Operations/Bitwise Operator  logicop=AND  UseBitMask=on  BitMask=65535  BitMaskRealWorld=Stored Integer
  MCU_HV_Voltage_O : Constant  Value=0  OutDataTypeStr=single
  MCU_HV_Voltage_S : ArithShift
  MCU_HV_Voltage_sat : Saturate  UpperLimit=1000  LowerLimit=0
  MCU_HV_Voltage_st : Sum  Inputs=+-
  MCU_HV_Voltageoutput8_C : Constant  Value=256
  output1 : Outport
  output2 : Outport  Port=2
  output3 : Outport  Port=3
  output4 : Outport  Port=4
  output5 : Outport  Port=5
  output6 : Outport  Port=6
  output7 : Outport  Port=7
  output8 : Outport  Port=8
  wires:
  MCU_HV_Voltage/1 -> MCU_HV_Voltage_sat/1
  MCU_HV_Voltage_sat/1 -> MCU_HV_Voltage_st/1
  MCU_HV_Voltage_O/1 -> MCU_HV_Voltage_st/2
  MCU_HV_Voltage_st/1 -> MCU_HV_Voltage_D/1
  MCU_HV_Voltage_F/1 -> MCU_HV_Voltage_D/2
  MCU_HV_Voltage_D/1 -> MCU_HV_VoltageRon/1
  MCU_HV_VoltageRon/1 -> MCU_HV_Voltage_S/1
  MCU_HV_Voltage_S/1 -> MCU_HV_Voltage_1sat/1
  MCU_HV_Voltage_1sat/1 -> MCU_HV_Voltage_Convert/1
  MCU_HV_Voltage_Convert/1 -> MCU_HV_Voltage_L/1
  MCU_HV_Voltage_L/1 -> MCU_HV_Voltage_D1/1, MCU_HV_Voltage_And/1
  MCU_HV_Voltageoutput8_C/1 -> MCU_HV_Voltage_D1/2
  MCU_HV_Voltage_D1/1 -> MCU_HV_VoltageCOV/1
  MCU_HV_VoltageCOV/1 -> output8/1
  MCU_HV_Voltage_And_C/1 -> MCU_HV_Voltage_And/2
  MCU_HV_Voltage_And/1 -> BitCov/1
  BitCov/1 -> output7/1
  Constant1/1 -> output1/1
  Constant2/1 -> output2/1
  Constant3/1 -> output3/1
  Constant4/1 -> output4/1
  Constant5/1 -> output5/1
  Constant6/1 -> output6/1

== system E33_VCU_simulink/Subsystem1/MCUctrl/VCU_MCU_CMD/MCU_IsBrakeMode ==
  MCU_IsBrakeMode : Inport
  Constant{1..4,6..8} (7 alike) : Constant  Value=0  OutDataTypeStr=uint8  SampleTime=-1
  MCU_IsBrakeModeRon : Rounding  Operator=round
  MCU_IsBrakeMode_1sat : Saturate  UpperLimit=8  LowerLimit=0
  MCU_IsBrakeMode_Convert : DataTypeConversion  OutDataTypeStr=uint8
  MCU_IsBrakeMode_Convert1 : DataTypeConversion  OutDataTypeStr=uint32
  MCU_IsBrakeMode_D : Product  Inputs=*/
  MCU_IsBrakeMode_F : Constant  OutDataTypeStr=single
  MCU_IsBrakeMode_L : simulink/Logic and Bit Operations/Bitwise Operator  logicop=AND  UseBitMask=on  BitMask=8  BitMaskRealWorld=Stored Integer
  MCU_IsBrakeMode_O : Constant  Value=0  OutDataTypeStr=single
  MCU_IsBrakeMode_S : ArithShift  BitShiftNumber=-3
  MCU_IsBrakeMode_sat : Saturate  UpperLimit=1  LowerLimit=0
  MCU_IsBrakeMode_st : Sum  Inputs=+-
  output1 : Outport
  output2 : Outport  Port=2
  output3 : Outport  Port=3
  output4 : Outport  Port=4
  output5 : Outport  Port=5
  output6 : Outport  Port=6
  output7 : Outport  Port=7
  output8 : Outport  Port=8
  wires:
  MCU_IsBrakeMode/1 -> MCU_IsBrakeMode_sat/1
  MCU_IsBrakeMode_sat/1 -> MCU_IsBrakeMode_st/1
  MCU_IsBrakeMode_O/1 -> MCU_IsBrakeMode_st/2
  MCU_IsBrakeMode_st/1 -> MCU_IsBrakeMode_D/1
  MCU_IsBrakeMode_F/1 -> MCU_IsBrakeMode_D/2
  MCU_IsBrakeMode_D/1 -> MCU_IsBrakeModeRon/1
  MCU_IsBrakeModeRon/1 -> MCU_IsBrakeMode_S/1
  MCU_IsBrakeMode_S/1 -> MCU_IsBrakeMode_1sat/1
  MCU_IsBrakeMode_1sat/1 -> MCU_IsBrakeMode_Convert1/1
  MCU_IsBrakeMode_Convert1/1 -> MCU_IsBrakeMode_L/1
  MCU_IsBrakeMode_L/1 -> MCU_IsBrakeMode_Convert/1
  MCU_IsBrakeMode_Convert/1 -> output5/1
  Constant1/1 -> output1/1
  Constant2/1 -> output2/1
  Constant3/1 -> output3/1
  Constant4/1 -> output4/1
  Constant6/1 -> output6/1
  Constant7/1 -> output7/1
  Constant8/1 -> output8/1

== system E33_VCU_simulink/Subsystem1/MCUctrl/VCU_MCU_CMD/MCU_IsFreeMode ==
  MCU_IsFreeMode : Inport
  Constant{1..4,6..8} (7 alike) : Constant  Value=0  OutDataTypeStr=uint8  SampleTime=-1
  MCU_IsFreeModeRon : Rounding  Operator=round
  MCU_IsFreeMode_1sat : Saturate  UpperLimit=1  LowerLimit=0
  MCU_IsFreeMode_Convert : DataTypeConversion  OutDataTypeStr=uint8
  MCU_IsFreeMode_Convert1 : DataTypeConversion  OutDataTypeStr=uint32
  MCU_IsFreeMode_D : Product  Inputs=*/
  MCU_IsFreeMode_F : Constant  OutDataTypeStr=single
  MCU_IsFreeMode_L : simulink/Logic and Bit Operations/Bitwise Operator  logicop=AND  UseBitMask=on  BitMask=1  BitMaskRealWorld=Stored Integer
  MCU_IsFreeMode_O : Constant  Value=0  OutDataTypeStr=single
  MCU_IsFreeMode_S : ArithShift
  MCU_IsFreeMode_sat : Saturate  UpperLimit=1  LowerLimit=0
  MCU_IsFreeMode_st : Sum  Inputs=+-
  output1 : Outport
  output2 : Outport  Port=2
  output3 : Outport  Port=3
  output4 : Outport  Port=4
  output5 : Outport  Port=5
  output6 : Outport  Port=6
  output7 : Outport  Port=7
  output8 : Outport  Port=8
  wires:
  MCU_IsFreeMode/1 -> MCU_IsFreeMode_sat/1
  MCU_IsFreeMode_sat/1 -> MCU_IsFreeMode_st/1
  MCU_IsFreeMode_O/1 -> MCU_IsFreeMode_st/2
  MCU_IsFreeMode_st/1 -> MCU_IsFreeMode_D/1
  MCU_IsFreeMode_F/1 -> MCU_IsFreeMode_D/2
  MCU_IsFreeMode_D/1 -> MCU_IsFreeModeRon/1
  MCU_IsFreeModeRon/1 -> MCU_IsFreeMode_S/1
  MCU_IsFreeMode_S/1 -> MCU_IsFreeMode_1sat/1
  MCU_IsFreeMode_1sat/1 -> MCU_IsFreeMode_Convert1/1
  MCU_IsFreeMode_Convert1/1 -> MCU_IsFreeMode_L/1
  MCU_IsFreeMode_L/1 -> MCU_IsFreeMode_Convert/1
  MCU_IsFreeMode_Convert/1 -> output5/1
  Constant1/1 -> output1/1
  Constant2/1 -> output2/1
  Constant3/1 -> output3/1
  Constant4/1 -> output4/1
  Constant6/1 -> output6/1
  Constant7/1 -> output7/1
  Constant8/1 -> output8/1

== system E33_VCU_simulink/Subsystem1/MCUctrl/VCU_MCU_CMD/MCU_IsMcuNOTActive ==
  MCU_IsMcuNOTActive : Inport
  Constant{1..4,6..8} (7 alike) : Constant  Value=0  OutDataTypeStr=uint8  SampleTime=-1
  MCU_IsMcuNOTActiveRon : Rounding  Operator=round
  MCU_IsMcuNOTActive_1sat : Saturate  UpperLimit=128  LowerLimit=0
  MCU_IsMcuNOTActive_Convert : DataTypeConversion  OutDataTypeStr=uint8
  MCU_IsMcuNOTActive_Convert1 : DataTypeConversion  OutDataTypeStr=uint32
  MCU_IsMcuNOTActive_D : Product  Inputs=*/
  MCU_IsMcuNOTActive_F : Constant  OutDataTypeStr=single
  MCU_IsMcuNOTActive_L : simulink/Logic and Bit Operations/Bitwise Operator  logicop=AND  UseBitMask=on  BitMask=128  BitMaskRealWorld=Stored Integer
  MCU_IsMcuNOTActive_O : Constant  Value=0  OutDataTypeStr=single
  MCU_IsMcuNOTActive_S : ArithShift  BitShiftNumber=-7
  MCU_IsMcuNOTActive_sat : Saturate  UpperLimit=1  LowerLimit=0
  MCU_IsMcuNOTActive_st : Sum  Inputs=+-
  output1 : Outport
  output2 : Outport  Port=2
  output3 : Outport  Port=3
  output4 : Outport  Port=4
  output5 : Outport  Port=5
  output6 : Outport  Port=6
  output7 : Outport  Port=7
  output8 : Outport  Port=8
  wires:
  MCU_IsMcuNOTActive/1 -> MCU_IsMcuNOTActive_sat/1
  MCU_IsMcuNOTActive_sat/1 -> MCU_IsMcuNOTActive_st/1
  MCU_IsMcuNOTActive_O/1 -> MCU_IsMcuNOTActive_st/2
  MCU_IsMcuNOTActive_st/1 -> MCU_IsMcuNOTActive_D/1
  MCU_IsMcuNOTActive_F/1 -> MCU_IsMcuNOTActive_D/2
  MCU_IsMcuNOTActive_D/1 -> MCU_IsMcuNOTActiveRon/1
  MCU_IsMcuNOTActiveRon/1 -> MCU_IsMcuNOTActive_S/1
  MCU_IsMcuNOTActive_S/1 -> MCU_IsMcuNOTActive_1sat/1
  MCU_IsMcuNOTActive_1sat/1 -> MCU_IsMcuNOTActive_Convert1/1
  MCU_IsMcuNOTActive_Convert1/1 -> MCU_IsMcuNOTActive_L/1
  MCU_IsMcuNOTActive_L/1 -> MCU_IsMcuNOTActive_Convert/1
  MCU_IsMcuNOTActive_Convert/1 -> output5/1
  Constant1/1 -> output1/1
  Constant2/1 -> output2/1
  Constant3/1 -> output3/1
  Constant4/1 -> output4/1
  Constant6/1 -> output6/1
  Constant7/1 -> output7/1
  Constant8/1 -> output8/1

== system E33_VCU_simulink/Subsystem1/MCUctrl/VCU_MCU_CMD/MCU_IsPosRelayAct ==
  MCU_IsPosRelayAct : Inport
  Constant{1..5,7..8} (7 alike) : Constant  Value=0  OutDataTypeStr=uint8  SampleTime=-1
  MCU_IsPosRelayActRon : Rounding  Operator=round
  MCU_IsPosRelayAct_1sat : Saturate  UpperLimit=8  LowerLimit=0
  MCU_IsPosRelayAct_Convert : DataTypeConversion  OutDataTypeStr=uint8
  MCU_IsPosRelayAct_Convert1 : DataTypeConversion  OutDataTypeStr=uint32
  MCU_IsPosRelayAct_D : Product  Inputs=*/
  MCU_IsPosRelayAct_F : Constant  OutDataTypeStr=single
  MCU_IsPosRelayAct_L : simulink/Logic and Bit Operations/Bitwise Operator  logicop=AND  UseBitMask=on  BitMask=8  BitMaskRealWorld=Stored Integer
  MCU_IsPosRelayAct_O : Constant  Value=0  OutDataTypeStr=single
  MCU_IsPosRelayAct_S : ArithShift  BitShiftNumber=-3
  MCU_IsPosRelayAct_sat : Saturate  UpperLimit=1  LowerLimit=0
  MCU_IsPosRelayAct_st : Sum  Inputs=+-
  output1 : Outport
  output2 : Outport  Port=2
  output3 : Outport  Port=3
  output4 : Outport  Port=4
  output5 : Outport  Port=5
  output6 : Outport  Port=6
  output7 : Outport  Port=7
  output8 : Outport  Port=8
  wires:
  MCU_IsPosRelayAct/1 -> MCU_IsPosRelayAct_sat/1
  MCU_IsPosRelayAct_sat/1 -> MCU_IsPosRelayAct_st/1
  MCU_IsPosRelayAct_O/1 -> MCU_IsPosRelayAct_st/2
  MCU_IsPosRelayAct_st/1 -> MCU_IsPosRelayAct_D/1
  MCU_IsPosRelayAct_F/1 -> MCU_IsPosRelayAct_D/2
  MCU_IsPosRelayAct_D/1 -> MCU_IsPosRelayActRon/1
  MCU_IsPosRelayActRon/1 -> MCU_IsPosRelayAct_S/1
  MCU_IsPosRelayAct_S/1 -> MCU_IsPosRelayAct_1sat/1
  MCU_IsPosRelayAct_1sat/1 -> MCU_IsPosRelayAct_Convert1/1
  MCU_IsPosRelayAct_Convert1/1 -> MCU_IsPosRelayAct_L/1
  MCU_IsPosRelayAct_L/1 -> MCU_IsPosRelayAct_Convert/1
  MCU_IsPosRelayAct_Convert/1 -> output6/1
  Constant1/1 -> output1/1
  Constant2/1 -> output2/1
  Constant3/1 -> output3/1
  Constant4/1 -> output4/1
  Constant5/1 -> output5/1
  Constant7/1 -> output7/1
  Constant8/1 -> output8/1

== system E33_VCU_simulink/Subsystem1/MCUctrl/VCU_MCU_CMD/MCU_IsSpdMode ==
  MCU_IsSpdMode : Inport
  Constant{1..4,6..8} (7 alike) : Constant  Value=0  OutDataTypeStr=uint8  SampleTime=-1
  MCU_IsSpdModeRon : Rounding  Operator=round
  MCU_IsSpdMode_1sat : Saturate  UpperLimit=4  LowerLimit=0
  MCU_IsSpdMode_Convert : DataTypeConversion  OutDataTypeStr=uint8
  MCU_IsSpdMode_Convert1 : DataTypeConversion  OutDataTypeStr=uint32
  MCU_IsSpdMode_D : Product  Inputs=*/
  MCU_IsSpdMode_F : Constant  OutDataTypeStr=single
  MCU_IsSpdMode_L : simulink/Logic and Bit Operations/Bitwise Operator  logicop=AND  UseBitMask=on  BitMask=4  BitMaskRealWorld=Stored Integer
  MCU_IsSpdMode_O : Constant  Value=0  OutDataTypeStr=single
  MCU_IsSpdMode_S : ArithShift  BitShiftNumber=-2
  MCU_IsSpdMode_sat : Saturate  UpperLimit=1  LowerLimit=0
  MCU_IsSpdMode_st : Sum  Inputs=+-
  output1 : Outport
  output2 : Outport  Port=2
  output3 : Outport  Port=3
  output4 : Outport  Port=4
  output5 : Outport  Port=5
  output6 : Outport  Port=6
  output7 : Outport  Port=7
  output8 : Outport  Port=8
  wires:
  MCU_IsSpdMode/1 -> MCU_IsSpdMode_sat/1
  MCU_IsSpdMode_sat/1 -> MCU_IsSpdMode_st/1
  MCU_IsSpdMode_O/1 -> MCU_IsSpdMode_st/2
  MCU_IsSpdMode_st/1 -> MCU_IsSpdMode_D/1
  MCU_IsSpdMode_F/1 -> MCU_IsSpdMode_D/2
  MCU_IsSpdMode_D/1 -> MCU_IsSpdModeRon/1
  MCU_IsSpdModeRon/1 -> MCU_IsSpdMode_S/1
  MCU_IsSpdMode_S/1 -> MCU_IsSpdMode_1sat/1
  MCU_IsSpdMode_1sat/1 -> MCU_IsSpdMode_Convert1/1
  MCU_IsSpdMode_Convert1/1 -> MCU_IsSpdMode_L/1
  MCU_IsSpdMode_L/1 -> MCU_IsSpdMode_Convert/1
  MCU_IsSpdMode_Convert/1 -> output5/1
  Constant1/1 -> output1/1
  Constant2/1 -> output2/1
  Constant3/1 -> output3/1
  Constant4/1 -> output4/1
  Constant6/1 -> output6/1
  Constant7/1 -> output7/1
  Constant8/1 -> output8/1

== system E33_VCU_simulink/Subsystem1/MCUctrl/VCU_MCU_CMD/MCU_IsTorqMode ==
  MCU_IsTorqMode : Inport
  Constant{1..4,6..8} (7 alike) : Constant  Value=0  OutDataTypeStr=uint8  SampleTime=-1
  MCU_IsTorqModeRon : Rounding  Operator=round
  MCU_IsTorqMode_1sat : Saturate  UpperLimit=2  LowerLimit=0
  MCU_IsTorqMode_Convert : DataTypeConversion  OutDataTypeStr=uint8
  MCU_IsTorqMode_Convert1 : DataTypeConversion  OutDataTypeStr=uint32
  MCU_IsTorqMode_D : Product  Inputs=*/
  MCU_IsTorqMode_F : Constant  OutDataTypeStr=single
  MCU_IsTorqMode_L : simulink/Logic and Bit Operations/Bitwise Operator  logicop=AND  UseBitMask=on  BitMask=2  BitMaskRealWorld=Stored Integer
  MCU_IsTorqMode_O : Constant  Value=0  OutDataTypeStr=single
  MCU_IsTorqMode_S : ArithShift  BitShiftNumber=-1
  MCU_IsTorqMode_sat : Saturate  UpperLimit=1  LowerLimit=0
  MCU_IsTorqMode_st : Sum  Inputs=+-
  output1 : Outport
  output2 : Outport  Port=2
  output3 : Outport  Port=3
  output4 : Outport  Port=4
  output5 : Outport  Port=5
  output6 : Outport  Port=6
  output7 : Outport  Port=7
  output8 : Outport  Port=8
  wires:
  MCU_IsTorqMode/1 -> MCU_IsTorqMode_sat/1
  MCU_IsTorqMode_sat/1 -> MCU_IsTorqMode_st/1
  MCU_IsTorqMode_O/1 -> MCU_IsTorqMode_st/2
  MCU_IsTorqMode_st/1 -> MCU_IsTorqMode_D/1
  MCU_IsTorqMode_F/1 -> MCU_IsTorqMode_D/2
  MCU_IsTorqMode_D/1 -> MCU_IsTorqModeRon/1
  MCU_IsTorqModeRon/1 -> MCU_IsTorqMode_S/1
  MCU_IsTorqMode_S/1 -> MCU_IsTorqMode_1sat/1
  MCU_IsTorqMode_1sat/1 -> MCU_IsTorqMode_Convert1/1
  MCU_IsTorqMode_Convert1/1 -> MCU_IsTorqMode_L/1
  MCU_IsTorqMode_L/1 -> MCU_IsTorqMode_Convert/1
  MCU_IsTorqMode_Convert/1 -> output5/1
  Constant1/1 -> output1/1
  Constant2/1 -> output2/1
  Constant3/1 -> output3/1
  Constant4/1 -> output4/1
  Constant6/1 -> output6/1
  Constant7/1 -> output7/1
  Constant8/1 -> output8/1

== system E33_VCU_simulink/Subsystem1/MCUctrl/VCU_MCU_CMD/MCU_IsZeroLocMode ==
  MCU_IsZeroLocMode : Inport
  Constant{1..4,6..8} (7 alike) : Constant  Value=0  OutDataTypeStr=uint8  SampleTime=-1
  MCU_IsZeroLocModeRon : Rounding  Operator=round
  MCU_IsZeroLocMode_1sat : Saturate  UpperLimit=16  LowerLimit=0
  MCU_IsZeroLocMode_Convert : DataTypeConversion  OutDataTypeStr=uint8
  MCU_IsZeroLocMode_Convert1 : DataTypeConversion  OutDataTypeStr=uint32
  MCU_IsZeroLocMode_D : Product  Inputs=*/
  MCU_IsZeroLocMode_F : Constant  OutDataTypeStr=single
  MCU_IsZeroLocMode_L : simulink/Logic and Bit Operations/Bitwise Operator  logicop=AND  UseBitMask=on  BitMask=16  BitMaskRealWorld=Stored Integer
  MCU_IsZeroLocMode_O : Constant  Value=0  OutDataTypeStr=single
  MCU_IsZeroLocMode_S : ArithShift  BitShiftNumber=-4
  MCU_IsZeroLocMode_sat : Saturate  UpperLimit=1  LowerLimit=0
  MCU_IsZeroLocMode_st : Sum  Inputs=+-
  output1 : Outport
  output2 : Outport  Port=2
  output3 : Outport  Port=3
  output4 : Outport  Port=4
  output5 : Outport  Port=5
  output6 : Outport  Port=6
  output7 : Outport  Port=7
  output8 : Outport  Port=8
  wires:
  MCU_IsZeroLocMode/1 -> MCU_IsZeroLocMode_sat/1
  MCU_IsZeroLocMode_sat/1 -> MCU_IsZeroLocMode_st/1
  MCU_IsZeroLocMode_O/1 -> MCU_IsZeroLocMode_st/2
  MCU_IsZeroLocMode_st/1 -> MCU_IsZeroLocMode_D/1
  MCU_IsZeroLocMode_F/1 -> MCU_IsZeroLocMode_D/2
  MCU_IsZeroLocMode_D/1 -> MCU_IsZeroLocModeRon/1
  MCU_IsZeroLocModeRon/1 -> MCU_IsZeroLocMode_S/1
  MCU_IsZeroLocMode_S/1 -> MCU_IsZeroLocMode_1sat/1
  MCU_IsZeroLocMode_1sat/1 -> MCU_IsZeroLocMode_Convert1/1
  MCU_IsZeroLocMode_Convert1/1 -> MCU_IsZeroLocMode_L/1
  MCU_IsZeroLocMode_L/1 -> MCU_IsZeroLocMode_Convert/1
  MCU_IsZeroLocMode_Convert/1 -> output5/1
  Constant1/1 -> output1/1
  Constant2/1 -> output2/1
  Constant3/1 -> output3/1
  Constant4/1 -> output4/1
  Constant6/1 -> output6/1
  Constant7/1 -> output7/1
  Constant8/1 -> output8/1
